simulink model "ModelVls"  (R2022b)
settings: Solver=FixedStepDiscrete  StartTime=0.0  StopTime=1  RelTol=1e-3  EnableMultiTasking=on
InitFcn:
  | % Initialize model
  | run([ModelRootName() 'Init.m']);
  | 
  | % load library data
  | GainLibrary_data;
StartFcn:
  | % make sure all the simulated RTC requests are found
  | %RTC_SIM_OBJ.ValidateREQs();
model workspace (MAT data in the model file):
  PreampVolumeTable_Idx : Simulink.Signal (value not decoded)
  Range : Simulink.Signal (value not decoded)
  Table_Idx : Simulink.Signal (value not decoded)
undefined symbols (not defined in the file): Config, Ifir, IFIR, MedusaConfig, MuteRamper, MuteRamperBtc, numAudioIn, preAmp, Row, sys_defs, VLSConfig
libraries: FeaturePath x22, TuneVar x17, RTC x9, MedusaDelays x9, dspindex x5, TOP x5, SampleRateConverter x4, EdgePorts x2, PooliirLib x2, MedusaCaeEnable x2, FIREven x2, VLSGains x2
(part 3 of 4)

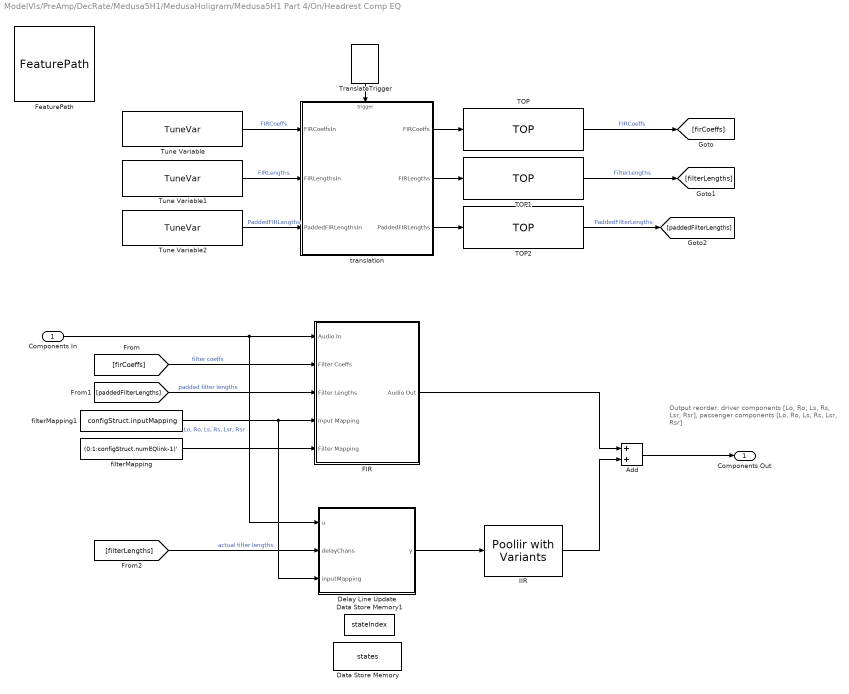
== system ModelVls/PreAmp/DecRate/Medusa5H1/MedusaHoligram/Medusa5H1 Part 4/On/Headrest Comp EQ ==
  note: Output reorder:
      | driver components [Lo, Ro, Ls, Rs, Lsr, Rsr],
      | passenger components [Lo, Ro, Ls, Rs, Lsr, Rsr]
  Components In : Inport
  Add : Sum  Priority=2
  Data Store Memory : DataStoreMemory  DataStoreName=states  ReadBeforeWriteMsg=warning  WriteAfterWriteMsg=warning  WriteAfterReadMsg=warning  InitialValue=zeros(fixedDelayLength, numInput)  ShowAdditionalParam=off  OutDataTypeStr=single
  Data Store Memory1 : DataStoreMemory  DataStoreName=stateIndex  ReadBeforeWriteMsg=warning  WriteAfterWriteMsg=warning  WriteAfterReadMsg=warning  ShowAdditionalParam=off  OutDataTypeStr=int32
  Delay Line Update : MATLAB Function  TreatAsAtomicUnit=on
  FIR : Subsystem  AncestorBlock=FIRGeneric/Generic FIR  mask(FIR Generic){variantSelect=Hexagon, stateBufferSize=configStruct.totalBufferSize, numOut=configStruct.numEQlink, frameSize=0, numIn=0}
      mask prompts: variantSelect "Implementation:"; stateBufferSize "State buffer size:"; numOut "Number of outputs:"; frameSize "Frame size:"; numIn "Number of inputs:"
      mask help:
      | Generic FIR is a configurable multi-channel FIR filter that supports one or more channels.  Different filter coefficients and number of coefficients can be used for each channel filter.  There can be fewer inputs than outputs, with some inputs routed to more than one output filter.   Identical filter configurations can also be used for multiple output filters.  The Generic FIR model supports three different implementations, selectable from the model mask:
      |
      | (i)  Core: FIR filters executing on core with target specific CRL support
      | (ii) Accel: FIR filters executing on IIR hardware accelerator, offloading MIPS usage from core
      | (iii) Hexagon: FIR filters executing on Hexagon DSP
      | (iv) Generic: FIR filters executing on core without CRL support
      |
      | NOTE: The Generic FIR codeWorkMemory buffer should always be mapped to L1 memory or core MIPS usage will increase.
      |
      | For more information, please see 'Help'.
      mask init:
      | % Create alias for code work memory buffer for each instance of model
      | FirGenericMask(gcbh, variantSelect);
      | 
      | % There are three implementation types:
      | % Type    Value  Description
      | % CORE    1      Optimized assembly running on core
      | % ACCEL   2      Computing offloaded to accelerator peripheral
      | % HEXAGON 3      Optimized C/assembly code running on Hexagon DSP
      | % GENERIC 4      Generic implementation for other targets without CRL
      | 
      | if variantSelect == 1
      |     % 6 variable size arrays (for input, coeffs, states, 
      |     % stateSharingEnabled, taps array per output channel,
      |     % and mapped audio input offsets) 
      |     % + 10 struct members
      |     codeWorkMemorySize = numOut * 6 + 10;  % words
      |     
      | elseif variantSelect == 2
      |     % Accelerator CRL code work memory size is equal to:
      |     %             sizeof(accelWorkMemory_t) + variableDataSize;
      |     % with variable data size dependent on number inputs, number outputs
      |     % and frame size.  NOTE: this must be updated to match the CRL code
      |     % if any changes are made to the accelWorkMemory_t structure.
      |     codeWorkMemorySize = 156 + (24 + numIn*48 + numOut*40);  % bytes
      |     codeWorkMemorySize = codeWorkMemorySize / 4;  % words (single)
      | 
      | elseif variantSelect == 3    
      |     codeWorkMemorySize = 156 + (24 + numIn*8 + numOut*(80 + 4*frameSize));  % bytes
      |     codeWorkMemorySize = codeWorkMemorySize / 4;  % words (single)
      |     
      | else
      |     % This is not used if there is no CRL
      |     codeWorkMemorySize = 1;
      | end
      settings: LibrarySourceBlock=FIRGeneric/Generic FIR
      mask Help:
      | Generic multi-channel FIR block supports multiple inputs, outputs and coefficient sets. Some inputs may drive multiple outputs, and this input sharing is specified by an input mapping per output. Some filters may be shared among multiple outputs, and this filter sharing is specified by a filter mapping per output. Input sharing assumes all filters sharing the same input have the same length to support state buffer sharing.
      | 
      | <b>Input signals: </b>
      | u: input channels [frame size x number of inputs]
      | coeffs: coefficient sets [total sum of filter lengths x 1]
      | filterLengths: array of filter lengths [number of filters x 1]
      | inputMapping: zero-based input mapping for each output [number of outputs x 1]
      | filterMapping:  zero-based filter mapping for each output [number of outputs x 1]
      | 
      | <b>Output signals: </b>
      | y: output channels [frame size x number of outputs]
      | 
      | <b>Mask parameters: </b>
      | Implementation: Core/Accel /Generic
      | State buffer size: total size of state buffer [total state buffer size x 1]
      | Number of outputs
      | Frame size
      | Number of inputs
      mask TypeOptions variantSelect: Core | Accel | Hexagon | Generic
      mask Callback variantSelect:
      | % Get the mask parameter value
      | maskStr = get_param(gcb,'variantSelect');
      | 
      | % Check the value of 'variantSelect'
      | if (~strcmp(maskStr,"Accel"))
      |     % Turn the visibility of 'frameSize' and 'numChannels' OFF
      |     set_param(gcb,'MaskVisibilities',{'on';'on';'on';'off';'off'});
      | else
      |     % "Accel": Set the visibility of all parameters to ON
      |     set_param(gcb,'MaskVisibilities',{'on';'on';'on';'on';'on'});
      | end
  FeaturePath : FeaturePath/FeaturePath  FeatureName=HeadrestCompEQ  IsGroup=off  GroupNumber=-1  IsModule=off  TriggerInit=[175 204 290 311]
      settings: SourceProductName=Bose Talaria
  IIR : PooliirAccel/Pooliir with Variants  variantSelect=Hexagon  maxNumStages=IIR.maxNumStages  numStages=IIR.numStages  sosCoefficients=IIR.coeffs  frameSize=0  numChannels=0  FeatureName=IIR
  TOP : TOP/TOP  TriggerInit=[815 320 985 380]  TopName=FIRCoeffs  DataType=single  BankNumber=1  PreOverlay=false  PostOverlay=false  Role=Automatic
      settings: SourceProductName=Bose Talaria
  TOP1 : TOP/TOP  TriggerInit=[815 390 985 450]  TopName=FilterLengths  DataType=uint32  BankNumber=0  PreOverlay=false  PostOverlay=false  Role=Automatic
      settings: SourceProductName=Bose Talaria
  TOP2 : TOP/TOP  TriggerInit=[815 460 985 520]  TopName=PaddedFilterLengths  DataType=uint32  BankNumber=0  PreOverlay=false  PostOverlay=false  Role=Automatic
      settings: SourceProductName=Bose Talaria
  TranslateTrigger : TuneVar/TranslateTrigger  TriggerInit=[656 230 694 285]
      settings: SourceProductName=Bose Talaria
  Tune Variable : TuneVar/TuneVar  TuneName=FIRCoeffs  SpecifyMaxSize=off  VariableDim=1 (Row)  MaxSize=[firLength*numEQlink 1]  TunabilityNumber=1  MinValue=[]  MaxValue=[]  TriggerInit=[330 325 500 375]  MaskValue=firCoeffsDefault
      settings: SourceProductName=Bose Talaria
  Tune Variable1 : TuneVar/TuneVar  TuneName=FIRLengths  SpecifyMaxSize=off  VariableDim=1 (Row)  MaxSize=[1 1]  TunabilityNumber=1  MinValue=[]  MaxValue=[]  TriggerInit=[330 395 500 445]  MaskValue=firLength*ones(numEQlink,1)
      settings: SourceProductName=Bose Talaria
  Tune Variable2 : TuneVar/TuneVar  TuneName=PaddedFIRLengths  SpecifyMaxSize=off  VariableDim=1 (Row)  MaxSize=[1 1]  TunabilityNumber=1  MinValue=[]  MaxValue=[]  TriggerInit=[330 465 500 515]  MaskValue=firLength*ones(numEQlink,1)
      settings: SourceProductName=Bose Talaria
  filterMapping : Constant  Value=(0:1:configStruct.numEQlink-1)'  VectorParams1D=off  OutDataTypeStr=uint32
  filterMapping1 : Constant  Value=configStruct.inputMapping  VectorParams1D=off  OutDataTypeStr=uint32
  translation : MATLAB Function  TreatAsAtomicUnit=on
  Components Out : Outport  VectorParamsAs1DForOutWhenUnconnected=off
  wires:
  Add/1 -> Components Out/1
  [firCoeffs] -> FIR/2(Filter Coeffs)  "filter coeffs"
  FIR/1(Audio Out) -> Add/1
  translation/2(FIRLengths) -> TOP1/1
  IIR/1 -> Add/2
  Tune Variable1/1 -> translation/2(FIRLengthsIn)  "FIRLengths"
  TOP/1 -> [firCoeffs]  "FIRCoeffs"
  filterMapping/1 -> FIR/5(Filter Mapping)
  translation/1(FIRCoeffs) -> TOP/1
  Delay Line Update/1(y) -> IIR/1
  TranslateTrigger/1 -> translation/Trigger
  Tune Variable/1 -> translation/1(FIRCoeffsIn)  "FIRCoeffs"
  filterMapping1/1 -> FIR/4(Input Mapping), Delay Line Update/3(inputMapping)
  [paddedFilterLengths] -> FIR/3(Filter Lengths)  "padded filter lengths"
  TOP1/1 -> [filterLengths]  "FilterLengths"
  Components In/1 -> FIR/1(Audio In), Delay Line Update/1(u)  "Lo, Ro, Ls, Rs, Lsr, Rsr"
  Tune Variable2/1 -> translation/3(PaddedFIRLengthsIn)  "PaddedFIRLengths"
  TOP2/1 -> [paddedFilterLengths]  "PaddedFilterLengths"
  translation/3(PaddedFIRLengths) -> TOP2/1
  [filterLengths] -> Delay Line Update/2(delayChans)  "actual filter lengths"

== system ModelVls/PreAmp/DecRate/Medusa5H1/PreAmpPart2/MuteRamperDR/InnerLink/Ramping_Subsystem ==
  audioIn : Inport
  Cg : Inport  Port=2
  Tg : Inport  Port=3
  RampCoeffs : Inport  Port=4
  SnapThresh : Inport  Port=5
  RampingGain : Subsystem
  Variable Selector : dspindex/Variable Selector  NumInputs=1  rowsOrCols=Rows  IdxMode=Fixed  Elements=Config.SamplesPerFrame  ZerOneIdxMode=One-based  errmode=Clip Index  FillMode=on  FillValues=0
  applyGain : Subsystem
  Out : Outport  VectorParamsAs1DForOutWhenUnconnected=off
  current_gain : Outport  Port=2  VectorParamsAs1DForOutWhenUnconnected=off
  wires:
  RampCoeffs/1 -> RampingGain/3(RampCoeffs)
  Tg/1 -> RampingGain/2(TargetGain)
  SnapThresh/1 -> RampingGain/4(SnapThresh)
  Cg/1 -> RampingGain/1(CurrentGain)
  Variable Selector/1 -> current_gain/1
  applyGain/1(Out1) -> Out/1
  audioIn/1 -> applyGain/2(In2)
  RampingGain/1(current_gain_out) -> Variable Selector/1, applyGain/1(In1)

== system ModelVls/PreAmp/DecRate/Medusa5H1/PreAmpPart2/MuteRamperFR/InnerLink/Ramping_Subsystem ==
  audioIn : Inport
  Cg : Inport  Port=2
  Tg : Inport  Port=3
  RampCoeffs : Inport  Port=4
  SnapThresh : Inport  Port=5
  RampingGain : Subsystem
  Variable Selector : dspindex/Variable Selector  NumInputs=1  rowsOrCols=Rows  IdxMode=Fixed  Elements=Config.SamplesPerFrame  ZerOneIdxMode=One-based  errmode=Clip Index  FillMode=on  FillValues=0
  applyGain : Subsystem
  Out : Outport  VectorParamsAs1DForOutWhenUnconnected=off
  current_gain : Outport  Port=2  VectorParamsAs1DForOutWhenUnconnected=off
  wires:
  RampCoeffs/1 -> RampingGain/3(RampCoeffs)
  Tg/1 -> RampingGain/2(TargetGain)
  SnapThresh/1 -> RampingGain/4(SnapThresh)
  Cg/1 -> RampingGain/1(CurrentGain)
  Variable Selector/1 -> current_gain/1
  applyGain/1(Out1) -> Out/1
  audioIn/1 -> applyGain/2(In2)
  RampingGain/1(current_gain_out) -> Variable Selector/1, applyGain/1(In1)

== system ModelVls/PreAmp/DecRate/Medusa5H1/MedusaHoligram/Medusa5H1 Part 3/On/SLC/Merge NTF_done ==
  NTF_done_DR : Inport
  NTF_done_FR : Inport  Port=2
  NTF_done_DR_VLS : Inport  Port=3
  NTF_done_FR_VLS : Inport  Port=4
  Trigger : TriggerPort  TriggerType=function-call  VariantControl=Variant  PortDimensions=1
  AND : Logic  Inputs=4  IconShape=distinctive  AllPortsSameDT=off  OutDataTypeStr=boolean
  NTF_done : Outport  VectorParamsAs1DForOutWhenUnconnected=off
  wires:
  NTF_done_FR_VLS/1 -> AND/4
  NTF_done_DR_VLS/1 -> AND/3
  NTF_done_DR/1 -> AND/1
  NTF_done_FR/1 -> AND/2
  AND/1 -> NTF_done/1

== system ModelVls/PreAmp/DecRate/Medusa5H1/MedusaHoligram/Medusa5H1 Part 4/On/Headrest Comp EQ/FIR ==
  Audio In : Inport
  Filter Coeffs : Inport  Port=2
  Filter Lengths : Inport  Port=3
  Input Mapping : Inport  Port=4
  Filter Mapping : Inport  Port=5
  FIR generic init : MATLAB Function  TreatAsAtomicUnit=on  RTWFcnName=foo
  FeaturePath : FeaturePath/FeaturePath  FeatureName=FIR  IsGroup=off  GroupNumber=-1  IsModule=off  TriggerInit=[105 -141 220 -34]
      settings: SourceProductName=Bose Talaria
  ITC : Subsystem  mask(Bose Initialization Trigger Control){}
      mask help: This block emits a function trigger for logic intended to execute at subsystem initialization time. Make sure not to reference any "live" signals
      mask init:
      | CodeID = InitTriggerControlMask.DoInit(gcbh);
      | ok = true;
      mask Display:
      | % retrieve icon definition
      | [path,w,h] = InitTriggerControlMask.Icon();
      | 
      | % retrieve the block's pixel size
      | pos = get(gcbh,'position');
      | bw = pos(3) - pos(1);
      | bh = pos(4) - pos(2);
      | 
      | % draw  icon to the center left
      | xAdj = bw/2 - w/2;
      | yAdj = bh/2 - h/2 + 4;
      | for i=1:length(path)
      |     patch(path(i).x+xAdj, path(i).y+yAdj, path(i).rgb);
      | end
      | 
      | text(bw*0.5, bh*0.2, 'ITC', 'horizontalAlignment', 'center');
      | 
      | % show X on error
      | if (exist('ok','var') && ok)
      | 	patch(0,0,[1 1 1]);
      | 	patch(bw,bh,[1 1 1]);
      | else
      | 	tx=bw*0.03;
      | 	ty=bh*0.03;
      | 	patch([0 tx bw bw-tx], [ty 0 bh-ty bh], [1 0 0]);
      | 	patch([0 bw-tx bw tx], [bh-ty 0 ty bh], [1 0 0]);
      | end
  MATLAB Function : MATLAB Function  TreatAsAtomicUnit=on
  codeWorkMemory : DataStoreMemory  DataStoreName=codeWorkMemory  WriteAfterWriteMsg=warning  InitialValue=zeros(1,codeWorkMemorySize)  ShowAdditionalParam=off  OutDataTypeStr=uint32
  stateBuffer : DataStoreMemory  DataStoreName=states  ReadBeforeWriteMsg=warning  WriteAfterWriteMsg=warning  WriteAfterReadMsg=warning  InitialValue=zeros(stateBufferSize,1)  ShowAdditionalParam=off  OutDataTypeStr=single
  Audio Out : Outport  VectorParamsAs1DForOutWhenUnconnected=off
  wires:
  Audio In/1 -> MATLAB Function/1(u), FIR generic init/1(u)
  ITC/1(Out1) -> FIR generic init/Trigger
  MATLAB Function/1(y) -> Audio Out/1
  Filter Mapping/1 -> MATLAB Function/5(filterMapping), FIR generic init/5(filterMapping)
  Filter Coeffs/1 -> MATLAB Function/2(coeffs), FIR generic init/2(coeffs)
  Input Mapping/1 -> MATLAB Function/4(inputMapping), FIR generic init/4(inputMapping)
  Filter Lengths/1 -> MATLAB Function/3(filterLengths), FIR generic init/3(filterLengths)

== system ModelVls/PreAmp/DecRate/Medusa5H1/PreAmpPart2/MuteRamperDR/InnerLink/Ramping_Subsystem/RampingGain ==
  CurrentGain : Inport
  TargetGain : Inport  Port=2
  RampCoeffs : Inport  Port=3
  SnapThresh : Inport  Port=4
  Abs3 : Abs  SaturateOnIntegerOverflow=off
  Add : Sum  Inputs=+-
  If : If  NumInputs=3  IfExpression=(u1>u2) & (u3>0)
  Max : MinMax  Function=max  Inputs=2
  Merge : Merge
  elseActionSubsystem : Subsystem
  frames : DataStoreRead  DataStoreName=nFrames  IndexOptions=Index vector (dialog)  Indices=1  OutputSizes=1
  ifActionSubsystem : Subsystem
  minGain : Constant  Value=Config.SilentGainLinear  OutDataTypeStr=single
  current_gain_out : Outport  VectorParamsAs1DForOutWhenUnconnected=off
  wires:
  frames/1 -> If/3, ifActionSubsystem/4(nFrames)
  elseActionSubsystem/1(Out1) -> Merge/2
  ifActionSubsystem/1(Out1) -> Merge/1
  RampCoeffs/1 -> ifActionSubsystem/1(rampCoeff)
  If/2 -> elseActionSubsystem/Action
  If/1 -> ifActionSubsystem/Action
  CurrentGain/1 -> Max/1
  minGain/1 -> Max/2
  Abs3/1 -> If/1
  SnapThresh/1 -> If/2
  TargetGain/1 -> elseActionSubsystem/1(In1), Add/1, ifActionSubsystem/2(TargetGain)
  Add/1 -> Abs3/1
  Merge/1 -> current_gain_out/1
  Max/1 -> Add/2, ifActionSubsystem/3(CurrentGain)

== system ModelVls/PreAmp/DecRate/Medusa5H1/PreAmpPart2/MuteRamperDR/InnerLink/Ramping_Subsystem/applyGain ==
  In1 : Inport
  In2 : Inport  Port=2
  For Each Subsystem : Subsystem  TreatAsAtomicUnit=on
  Out1 : Outport  VectorParamsAs1DForOutWhenUnconnected=off
  wires:
  In1/1 -> For Each Subsystem/1(In1)
  For Each Subsystem/1(Out1) -> Out1/1
  In2/1 -> For Each Subsystem/2(In2)

== system ModelVls/PreAmp/DecRate/Medusa5H1/PreAmpPart2/MuteRamperFR/InnerLink/Ramping_Subsystem/RampingGain ==
  CurrentGain : Inport
  TargetGain : Inport  Port=2
  RampCoeffs : Inport  Port=3
  SnapThresh : Inport  Port=4
  Abs3 : Abs  SaturateOnIntegerOverflow=off
  Add : Sum  Inputs=+-
  If : If  NumInputs=3  IfExpression=(u1>u2) & (u3>0)
  Max : MinMax  Function=max  Inputs=2
  Merge : Merge
  elseActionSubsystem : Subsystem
  frames : DataStoreRead  DataStoreName=nFrames  IndexOptions=Index vector (dialog)  Indices=1  OutputSizes=1
  ifActionSubsystem : Subsystem
  minGain : Constant  Value=Config.SilentGainLinear  OutDataTypeStr=single
  current_gain_out : Outport  VectorParamsAs1DForOutWhenUnconnected=off
  wires:
  frames/1 -> If/3, ifActionSubsystem/4(nFrames)
  elseActionSubsystem/1(Out1) -> Merge/2
  ifActionSubsystem/1(Out1) -> Merge/1
  RampCoeffs/1 -> ifActionSubsystem/1(rampCoeff)
  If/2 -> elseActionSubsystem/Action
  If/1 -> ifActionSubsystem/Action
  CurrentGain/1 -> Max/1
  minGain/1 -> Max/2
  Abs3/1 -> If/1
  SnapThresh/1 -> If/2
  TargetGain/1 -> elseActionSubsystem/1(In1), Add/1, ifActionSubsystem/2(TargetGain)
  Add/1 -> Abs3/1
  Merge/1 -> current_gain_out/1
  Max/1 -> Add/2, ifActionSubsystem/3(CurrentGain)

== system ModelVls/PreAmp/DecRate/Medusa5H1/PreAmpPart2/MuteRamperFR/InnerLink/Ramping_Subsystem/applyGain ==
  In1 : Inport
  In2 : Inport  Port=2
  For Each Subsystem : Subsystem  TreatAsAtomicUnit=on
  Out1 : Outport  VectorParamsAs1DForOutWhenUnconnected=off
  wires:
  In1/1 -> For Each Subsystem/1(In1)
  For Each Subsystem/1(Out1) -> Out1/1
  In2/1 -> For Each Subsystem/2(In2)

== system ModelVls/PreAmp/DecRate/Medusa5H1/MedusaHoligram/Medusa5H1 Part 4/On/Headrest Comp EQ/FIR/ITC ==
  ITC1 : S-Function  FunctionName=InitTriggerControl  Parameters=CodeID, 0  SFunctionDeploymentMode=off  EnableBusSupport=off
  init : MATLAB Function  TreatAsAtomicUnit=on  RTWFcnName=InitTrigger_Model_4079_595_209_62
      settings: RTWSystemCode=Nonreusable function
  Out1 : Outport  VectorParamsAs1DForOutWhenUnconnected=off
  wires:
  init/1(init()) -> Out1/1
  ITC1/1 -> init/Trigger

== system ModelVls/PreAmp/DecRate/Medusa5H1/PreAmpPart2/MuteRamperDR/InnerLink/Ramping_Subsystem/RampingGain/elseActionSubsystem ==
  In1 : Inport
  Action Port : ActionPort  ActionPortLabel=else
  Constant : Constant  Value=ones(Config.SamplesPerFrame,1)  VectorParams1D=off  OutDataTypeStr=single
  Multiply : Product
  Out1 : Outport  VectorParamsAs1DForOutWhenUnconnected=off
  wires:
  Constant/1 -> Multiply/1
  In1/1 -> Multiply/2
  Multiply/1 -> Out1/1

== system ModelVls/PreAmp/DecRate/Medusa5H1/PreAmpPart2/MuteRamperDR/InnerLink/Ramping_Subsystem/RampingGain/ifActionSubsystem ==
  note: IIR filter is used to get ramping up/down gain values. Filter transfer function
      |  is calculated for equation:
      | 	gain(n) = gain(n-1)*ramp_coeff
      |
      | Denominator coeff  = [1, -rampcoeff]  and Numerator coeff = 0
      | x0 : Initial state of the filter which is (currentGain * rampCoeff)
      | III : When target gain is updated through RTC, this signal will reset filter to
      | 	initial state to serve new RTC request
  rampCoeff : Inport
  TargetGain : Inport  Port=2
  CurrentGain : Inport  Port=3
  nFrames : Inport  Port=4
  Action Port : ActionPort  ActionPortLabel=if((u1>u2) & (u3>0))
  Add : Sum  Inputs=+-
  Constant : Constant  Value=ones(Config.SamplesPerFrame,1)  VectorParams1D=off  OutDataTypeStr=single
  Constant1 : Constant  OutDataTypeStr=single
  Data Store Write : DataStoreWrite  DataStoreName=nFrames  IndexOptions=Index vector (dialog)  Indices=1  OutputSizes=1
  Matrix Multiply : Product
  denCoefficient : Subsystem
  ramping_filter : DiscreteFilter  Numerator=0  DenominatorSource=Input port  Denominator=[1 -1.0003]  InitialStatesSource=Input port  InitialStates=1.0003  InputProcessing=Columns as channels (frame based)  ExternalReset=Level hold  FilterStructure=Direct form II transposed  a0EqualsOne=on
      settings: InputPortMap=u0,p3,r7,p5
  resetFilter : Subsystem
  Out1 : Outport
  wires:
  nFrames/1 -> Add/1
  Constant1/1 -> Add/2
  Add/1 -> Data Store Write/1
  Matrix Multiply/1 -> ramping_filter/4
  CurrentGain/1 -> Matrix Multiply/2
  ramping_filter/1 -> Out1/1
  Constant/1 -> ramping_filter/1
  rampCoeff/1 -> Matrix Multiply/1, denCoefficient/1(In1)
  resetFilter/1(Out1) -> ramping_filter/3
  denCoefficient/1(Out1) -> ramping_filter/2
  TargetGain/1 -> resetFilter/1(In1)

== system ModelVls/PreAmp/DecRate/Medusa5H1/PreAmpPart2/MuteRamperDR/InnerLink/Ramping_Subsystem/applyGain/For Each Subsystem ==
  In1 : Inport  Partition=on  PartitionDimension=1  PartitionWidth=1  PartitionOffset=0
  In2 : Inport  Port=2  Partition=on  PartitionDimension=1  PartitionWidth=1  PartitionOffset=0
  For Each : ForEach  DisableCoverage=on
  Multiply : Product  Multiplication=Matrix(*)
  Out1 : Outport  ConcatenationDimension=1
  wires:
  Multiply/1 -> Out1/1
  In2/1 -> Multiply/2
  In1/1 -> Multiply/1

== system ModelVls/PreAmp/DecRate/Medusa5H1/PreAmpPart2/MuteRamperFR/InnerLink/Ramping_Subsystem/RampingGain/elseActionSubsystem ==
  In1 : Inport
  Action Port : ActionPort  ActionPortLabel=else
  Constant : Constant  Value=ones(Config.SamplesPerFrame,1)  VectorParams1D=off  OutDataTypeStr=single
  Multiply : Product
  Out1 : Outport  VectorParamsAs1DForOutWhenUnconnected=off
  wires:
  Constant/1 -> Multiply/1
  In1/1 -> Multiply/2
  Multiply/1 -> Out1/1

== system ModelVls/PreAmp/DecRate/Medusa5H1/PreAmpPart2/MuteRamperFR/InnerLink/Ramping_Subsystem/RampingGain/ifActionSubsystem ==
  note: IIR filter is used to get ramping up/down gain values. Filter transfer function
      |  is calculated for equation:
      | 	gain(n) = gain(n-1)*ramp_coeff
      |
      | Denominator coeff  = [1, -rampcoeff]  and Numerator coeff = 0
      | x0 : Initial state of the filter which is (currentGain * rampCoeff)
      | III : When target gain is updated through RTC, this signal will reset filter to
      | 	initial state to serve new RTC request
  rampCoeff : Inport
  TargetGain : Inport  Port=2
  CurrentGain : Inport  Port=3
  nFrames : Inport  Port=4
  Action Port : ActionPort  ActionPortLabel=if((u1>u2) & (u3>0))
  Add : Sum  Inputs=+-
  Constant : Constant  Value=ones(Config.SamplesPerFrame,1)  VectorParams1D=off  OutDataTypeStr=single
  Constant1 : Constant  OutDataTypeStr=single
  Data Store Write : DataStoreWrite  DataStoreName=nFrames  IndexOptions=Index vector (dialog)  Indices=1  OutputSizes=1
  Matrix Multiply : Product
  denCoefficient : Subsystem
  ramping_filter : DiscreteFilter  Numerator=0  DenominatorSource=Input port  Denominator=[1 -1.0003]  InitialStatesSource=Input port  InitialStates=1.0003  InputProcessing=Columns as channels (frame based)  ExternalReset=Level hold  FilterStructure=Direct form II transposed  a0EqualsOne=on
      settings: InputPortMap=u0,p3,r7,p5
  resetFilter : Subsystem
  Out1 : Outport
  wires:
  nFrames/1 -> Add/1
  Constant1/1 -> Add/2
  Add/1 -> Data Store Write/1
  Matrix Multiply/1 -> ramping_filter/4
  CurrentGain/1 -> Matrix Multiply/2
  ramping_filter/1 -> Out1/1
  Constant/1 -> ramping_filter/1
  rampCoeff/1 -> Matrix Multiply/1, denCoefficient/1(In1)
  resetFilter/1(Out1) -> ramping_filter/3
  denCoefficient/1(Out1) -> ramping_filter/2
  TargetGain/1 -> resetFilter/1(In1)

== system ModelVls/PreAmp/DecRate/Medusa5H1/PreAmpPart2/MuteRamperFR/InnerLink/Ramping_Subsystem/applyGain/For Each Subsystem ==
  In1 : Inport  Partition=on  PartitionDimension=1  PartitionWidth=1  PartitionOffset=0
  In2 : Inport  Port=2  Partition=on  PartitionDimension=1  PartitionWidth=1  PartitionOffset=0
  For Each : ForEach  DisableCoverage=on
  Multiply : Product  Multiplication=Matrix(*)
  Out1 : Outport  ConcatenationDimension=1
  wires:
  Multiply/1 -> Out1/1
  In2/1 -> Multiply/2
  In1/1 -> Multiply/1

== system ModelVls/PreAmp/DecRate/Medusa5H1/PreAmpPart2/MuteRamperDR/InnerLink/Ramping_Subsystem/RampingGain/ifActionSubsystem/denCoefficient ==
  In1 : Inport
  Constant : Constant  Value=-1  OutDataTypeStr=single
  Constant3 : Constant  OutDataTypeStr=single
  Matrix Concatenate : Concatenate  Mode=Multidimensional array  ConcatenateDimension=2
  Multiply : Product
  Out1 : Outport  VectorParamsAs1DForOutWhenUnconnected=off
  wires:
  In1/1 -> Multiply/2
  Multiply/1 -> Matrix Concatenate/2
  Constant/1 -> Multiply/1
  Matrix Concatenate/1 -> Out1/1
  Constant3/1 -> Matrix Concatenate/1

== system ModelVls/PreAmp/DecRate/Medusa5H1/PreAmpPart2/MuteRamperDR/InnerLink/Ramping_Subsystem/RampingGain/ifActionSubsystem/resetFilter ==
  In1 : Inport
  Add2 : Sum  Inputs=+-
  Delay : Delay  DelayLength=1
  If : If  IfExpression=u1 == 0
  If Action Subsystem : Subsystem  TreatAsAtomicUnit=on
  If Action Subsystem1 : Subsystem  TreatAsAtomicUnit=on
  Merge : Merge
  Out1 : Outport  VectorParamsAs1DForOutWhenUnconnected=off
  wires:
  Merge/1 -> Out1/1
  If Action Subsystem1/1(Out1) -> Merge/2
  If Action Subsystem/1(Out1) -> Merge/1
  If/2 -> If Action Subsystem1/Action
  If/1 -> If Action Subsystem/Action
  In1/1 -> Delay/1, Add2/1
  Delay/1 -> Add2/2
  Add2/1 -> If/1

== system ModelVls/PreAmp/DecRate/Medusa5H1/PreAmpPart2/MuteRamperFR/InnerLink/Ramping_Subsystem/RampingGain/ifActionSubsystem/denCoefficient ==
  In1 : Inport
  Constant : Constant  Value=-1  OutDataTypeStr=single
  Constant3 : Constant  OutDataTypeStr=single
  Matrix Concatenate : Concatenate  Mode=Multidimensional array  ConcatenateDimension=2
  Multiply : Product
  Out1 : Outport  VectorParamsAs1DForOutWhenUnconnected=off
  wires:
  In1/1 -> Multiply/2
  Multiply/1 -> Matrix Concatenate/2
  Constant/1 -> Multiply/1
  Matrix Concatenate/1 -> Out1/1
  Constant3/1 -> Matrix Concatenate/1

== system ModelVls/PreAmp/DecRate/Medusa5H1/PreAmpPart2/MuteRamperFR/InnerLink/Ramping_Subsystem/RampingGain/ifActionSubsystem/resetFilter ==
  In1 : Inport
  Add2 : Sum  Inputs=+-
  Delay : Delay  DelayLength=1
  If : If  IfExpression=u1 == 0
  If Action Subsystem : Subsystem  TreatAsAtomicUnit=on
  If Action Subsystem1 : Subsystem  TreatAsAtomicUnit=on
  Merge : Merge
  Out1 : Outport  VectorParamsAs1DForOutWhenUnconnected=off
  wires:
  Merge/1 -> Out1/1
  If Action Subsystem1/1(Out1) -> Merge/2
  If Action Subsystem/1(Out1) -> Merge/1
  If/2 -> If Action Subsystem1/Action
  If/1 -> If Action Subsystem/Action
  In1/1 -> Delay/1, Add2/1
  Delay/1 -> Add2/2
  Add2/1 -> If/1

== system ModelVls/PreAmp/DecRate/Medusa5H1/PreAmpPart2/MuteRamperDR/InnerLink/Ramping_Subsystem/RampingGain/ifActionSubsystem/resetFilter/If Action Subsystem ==
  Action Port : ActionPort  ActionPortLabel=if(u1 == 0)
  Constant : Constant  Value=0  OutDataTypeStr=boolean
  Out1 : Outport  VectorParamsAs1DForOutWhenUnconnected=off
  wires:
  Constant/1 -> Out1/1

== system ModelVls/PreAmp/DecRate/Medusa5H1/PreAmpPart2/MuteRamperDR/InnerLink/Ramping_Subsystem/RampingGain/ifActionSubsystem/resetFilter/If Action Subsystem1 ==
  Action Port : ActionPort  ActionPortLabel=else
  Constant : Constant  OutDataTypeStr=boolean
  Out1 : Outport  VectorParamsAs1DForOutWhenUnconnected=off
  wires:
  Constant/1 -> Out1/1

== system ModelVls/PreAmp/DecRate/Medusa5H1/PreAmpPart2/MuteRamperFR/InnerLink/Ramping_Subsystem/RampingGain/ifActionSubsystem/resetFilter/If Action Subsystem ==
  Action Port : ActionPort  ActionPortLabel=if(u1 == 0)
  Constant : Constant  Value=0  OutDataTypeStr=boolean
  Out1 : Outport  VectorParamsAs1DForOutWhenUnconnected=off
  wires:
  Constant/1 -> Out1/1

== system ModelVls/PreAmp/DecRate/Medusa5H1/PreAmpPart2/MuteRamperFR/InnerLink/Ramping_Subsystem/RampingGain/ifActionSubsystem/resetFilter/If Action Subsystem1 ==
  Action Port : ActionPort  ActionPortLabel=else
  Constant : Constant  OutDataTypeStr=boolean
  Out1 : Outport  VectorParamsAs1DForOutWhenUnconnected=off
  wires:
  Constant/1 -> Out1/1

== matlab function ModelVls/PreAmp/DecRate/Medusa5H1/MedusaHoligram/Medusa5H1 Part 4/On/Headrest Comp EQ/translation ==
  data: FIRCoeffs output; FIRCoeffsIn input; FIRLengths output; FIRLengthsIn input; PaddedFIRLengthsIn input; PaddedFIRLengths output
  events: trigger input FUNCTION_CALL_EVENT
function [FIRCoeffs, FIRLengths, PaddedFIRLengths] = fcn(FIRCoeffsIn, FIRLengthsIn, PaddedFIRLengthsIn)

FIRCoeffs = FIRCoeffsIn.Value;
FIRLengths = FIRLengthsIn.Value;
PaddedFIRLengths = PaddedFIRLengthsIn.Value;

== matlab function ModelVls/PreAmp/DecRate/Medusa5H1/PreAmpPart2/MuteRamperDR/InnerLink/TriggeredFunction ==
  data: done output; targetLinearGain data_store_memory; currentGain data_store_memory
  events: trigger input FUNCTION_CALL_EVENT
function done = NotificationCheck()
% Function to check whether the ramp has completed. 
% If so, send out TRUE

global targetLinearGain;
global currentGain;

% Assume the work is complete until proven otherwise
done = true;
if (targetLinearGain ~= currentGain)
   done = false; % just proved otherwise
end

== matlab function ModelVls/PreAmp/DecRate/Medusa5H1/PreAmpPart2/MuteRamperDR/InnerLink/get_ramp_coeffs ==
  data: currentGainValue input; muteSwitch input; ramping_coeff output; rampingRate_dBPerSec input; rampingTime_ms input; Fs_Hz input; silentGainLinear parameter; targetLinearGain data_store_memory; nFrames data_store_memory; frameSize parameter
  events: trigger input FUNCTION_CALL_EVENT
function ramping_coeff = fcn(currentGainValue, muteSwitch, rampingRate_dBPerSec,rampingTime_ms, Fs_Hz, silentGainLinear, frameSize)

global targetLinearGain
global nFrames
targetLinearGain = single(1.0);

if muteSwitch
    targetLinearGain = single(max(0, silentGainLinear));
end

% % Nudge the gain values a bit if they are sitting at zero.
% % If current gain is zero, replace with a value very close to zero. What we
% % really want is a value which is on the edge of perception - not too small
% % or large. If the value is too small, we'll waste some of our ramp time
% % in perceived silence. If the value is too large, the audio will lurch
% % into perceptability at the start of the ramp.
% % So, 'max(currentGainValue, silentGainLinear)' & 'max(TargetGain, silentGainLinear)' are
% % used in equations

% In order to have the desired ramp time, the slope must vary dependent
% on the gain difference between target and current value.
% Equivalent ramp rate is therefore calculated as follows:

if (rampingRate_dBPerSec)
    currentGain_db = 20*log10(max(currentGainValue, silentGainLinear));
    targetGain_db = 20*log10( targetLinearGain);
    diff = abs(currentGain_db - targetGain_db);
    rampingTime_ms = diff / single(rampingRate_dBPerSec) * 1000;
end

quantum_ms = 1000 * frameSize / Fs_Hz;
numFrames = rampingTime_ms / quantum_ms;
% Do a ceil rather than a round to insure that we create enough
% frames. i.e. a fraction of a frame is promoted to an addition frame
nFrames = max (1, ceil(numFrames));
quantized_rampTime_ms = nFrames * quantum_ms;
   
% In order to have the desired ramp time, the slope must vary dependent
% on the gain differencebetween target and current value.
% Ramper's coefficient is therefore calculated as follows:
%
%   TargetGain = CurrentGain *( RampCoef ^ (Fs*RampTime_ms/1000) )
%
% therefore...
%
%                     log(TargetGain/CurrentGain)
%   log(RampCoef) = ------------------------------
%                        Fs*(RampTime_ms/1000)
%
ramping_coeff= exp(log( targetLinearGain /max(currentGainValue, silentGainLinear) ) / (Fs_Hz * quantized_rampTime_ms / 1000));

== matlab function ModelVls/PreAmp/DecRate/Medusa5H1/PreAmpPart2/MuteRamperFR/InnerLink/TriggeredFunction ==
  data: done output; targetLinearGain data_store_memory; currentGain data_store_memory
  events: trigger input FUNCTION_CALL_EVENT
function done = NotificationCheck()
% Function to check whether the ramp has completed. 
% If so, send out TRUE

global targetLinearGain;
global currentGain;

% Assume the work is complete until proven otherwise
done = true;
if (targetLinearGain ~= currentGain)
   done = false; % just proved otherwise
end

== matlab function ModelVls/PreAmp/DecRate/Medusa5H1/PreAmpPart2/MuteRamperFR/InnerLink/get_ramp_coeffs ==
  data: currentGainValue input; muteSwitch input; ramping_coeff output; rampingRate_dBPerSec input; rampingTime_ms input; Fs_Hz input; silentGainLinear parameter; targetLinearGain data_store_memory; nFrames data_store_memory; frameSize parameter
  events: trigger input FUNCTION_CALL_EVENT
function ramping_coeff = fcn(currentGainValue, muteSwitch, rampingRate_dBPerSec,rampingTime_ms, Fs_Hz, silentGainLinear, frameSize)

global targetLinearGain
global nFrames
targetLinearGain = single(1.0);

if muteSwitch
    targetLinearGain = single(max(0, silentGainLinear));
end

% % Nudge the gain values a bit if they are sitting at zero.
% % If current gain is zero, replace with a value very close to zero. What we
% % really want is a value which is on the edge of perception - not too small
% % or large. If the value is too small, we'll waste some of our ramp time
% % in perceived silence. If the value is too large, the audio will lurch
% % into perceptability at the start of the ramp.
% % So, 'max(currentGainValue, silentGainLinear)' & 'max(TargetGain, silentGainLinear)' are
% % used in equations

% In order to have the desired ramp time, the slope must vary dependent
% on the gain difference between target and current value.
% Equivalent ramp rate is therefore calculated as follows:

if (rampingRate_dBPerSec)
    currentGain_db = 20*log10(max(currentGainValue, silentGainLinear));
    targetGain_db = 20*log10( targetLinearGain);
    diff = abs(currentGain_db - targetGain_db);
    rampingTime_ms = diff / single(rampingRate_dBPerSec) * 1000;
end

quantum_ms = 1000 * frameSize / Fs_Hz;
numFrames = rampingTime_ms / quantum_ms;
% Do a ceil rather than a round to insure that we create enough
% frames. i.e. a fraction of a frame is promoted to an addition frame
nFrames = max (1, ceil(numFrames));
quantized_rampTime_ms = nFrames * quantum_ms;
   
% In order to have the desired ramp time, the slope must vary dependent
% on the gain differencebetween target and current value.
% Ramper's coefficient is therefore calculated as follows:
%
%   TargetGain = CurrentGain *( RampCoef ^ (Fs*RampTime_ms/1000) )
%
% therefore...
%
%                     log(TargetGain/CurrentGain)
%   log(RampCoef) = ------------------------------
%                        Fs*(RampTime_ms/1000)
%
ramping_coeff= exp(log( targetLinearGain /max(currentGainValue, silentGainLinear) ) / (Fs_Hz * quantized_rampTime_ms / 1000));

== matlab function ModelVls/PreAmp/DecRate/Medusa5H1/MedusaHoligram/Medusa5H1 Part 1/Medusa Band Split Stereo/Interpolated Filter/ifir ==
  data: audioIn input; coeffsFlip parameter; audioOut output; I parameter; states data_store_memory
function audioOut = ifir(audioIn, coeffsFlip, I)

% An interpolated FIR filter is an FIR filter with a sparse set of
% coefficients.  That is, the coefficients contain I-1 zeros between
% each point, so the effective length of  filter is len(input_coeffs) * I  
% The function support multiple channels, with each
% channel sharing the same set of filter coefficients.
% 
% p : coefficient set (non-zero coefficients)
% I : interpolation factor, I-1 zeros are inserted between each coefficient
% 
% NOTES: 
% The legacy IFIR block supported coefficient sets.  Currently
% this only supports one coefficient set. 
% The coefficients are stored flipped in time. The unflipped coeffs are
% passed to block mask, and the flipping is done in mask initialization.

% Initialize variables
[frameSize, numChannels] = size(audioIn);
[filterLength, ~] = size(coeffsFlip);

frameSize   = uint32(frameSize);
numChannels = uint32(numChannels);
filterLength = int32(filterLength);
activeCoeffSet = coder.const(uint32(zeros(1,numChannels)));

% State is a circular buffer that holds previous stateLen samples, 
% where state_index points to the last/oldest sample in the buffer, which 
% during processing will be overwritten by the current input sample.
global states;

persistent state_index;
if isempty(state_index)
    state_index = int32(0);
end

audioOut = IFIR(audioIn, frameSize, numChannels, states, filterLength, ...
                    state_index, coeffsFlip, activeCoeffSet, I);
                
end

function y = IFIR(audioIn, frameSize, numChannels, states2, filterLength, ...
                    state_index2, coeffsFlip, activeCoeffSet, I)
% If code gen'ing, generate warning if this is not replaced with IFIR.asm
%coder.replace('-warnifnoreplacement');

% We have to use a different state buffer and state index than the one 
% passed in.  Matlab value objects are passed by value, not by reference, 
% so the saving of states here does not work.  The state buffer and index 
% are still necessary to pass allocate in the calling function and pass 
% here in order to trigger CRL. This double buffering is annoying, however 
% only happens during simulation, not code generation. (taken from pooliir)
global states;
persistent state_index;
if isempty(state_index)
    state_index = int32(0);
end

y = coder.nullcopy(audioIn);
stateLen = filterLength * I;

for channel = 1:numChannels
    state = states(:,channel);
    stateIndex = state_index;
    coeffs = coeffsFlip(:,activeCoeffSet(channel)+1);
    
    for sample = 1:frameSize
        % overwrite oldest sample with the current input sample
        state(stateIndex+1) = audioIn(sample, channel);
        % go to the oldest sample (previously the 2nd oldest)
        stateIndex = stateIndex + I; 
        if (stateIndex >= stateLen)
            stateIndex = stateIndex - stateLen;
        end

        accum = single(0);
        for i = 1:filterLength
            accum = accum + (state(stateIndex+1) * coeffs(i));
            stateIndex = stateIndex + I; % skip zero coefficients
            if (stateIndex >= stateLen)
                    stateIndex = stateIndex - stateLen;
            end
        end
        y(sample, channel) = accum;

        % update stateIndex for next sample
        % because we subtract here state_index type is int32 not uint32
        stateIndex = stateIndex - (I-1);
        if (stateIndex < 0)
            stateIndex = stateIndex + stateLen;
        end
    end
 
    states(:, channel) = state;
end

state_index = stateIndex;

end

== matlab function ModelVls/NEAR/MATLAB Function ==
  data: u input; y output
function y = fcn(u)

y = u;

== matlab function ModelVls/PreAmp/Reset/MATLAB Function ==
  events: trigger input FUNCTION_CALL_EVENT
function fcn()

if coder.target('Rtw')
    coder.ceval('Model_Target_DRFDP_initialize');
    coder.ceval('Model_Target_FRFDP_initialize');
    coder.ceval('Model_Target_ExpandTailComponents_initialize');
    coder.ceval('Model_Target_TrebleandSurroundDelays_initialize');
    coder.ceval('Model_Target_Medusa5H1Part3_initialize');
    coder.ceval('Model_Target_Subsystem_initialize');
    
    coder.ceval('Model_Target_PreAmpPart1_Start');
    coder.ceval('Model_Target_SRCIn_Start');
%     coder.ceval('Model_Target_AudioPilot35_Start');
    coder.ceval('Model_Target_Medusa5H1Part1_Start');
    coder.ceval('Model_Target_Medusa5H1Part2_Start');
    coder.ceval('Model_Target_Medusa5H1Part3_Start');

    coder.ceval('Model_Target_PreAmpPart1_Init');
    coder.ceval('Model_Target_PreAmpPart2_Init');
%     coder.ceval('Model_Target_SRCIn_Init');
%     coder.ceval('Model_Target_SRCOut_Init');
%     coder.ceval('Model_Target_AudioPilot35_Init');
    coder.ceval('Model_Target_Medusa5H1Part1_Init');
    coder.ceval('Model_Target_Medusa5H1Part2_Init');
    coder.ceval('Model_Target_Medusa5H1Part3_Init');
end

== matlab function ModelVls/InputSelect/Reset/MATLAB Function ==
  events: trigger input FUNCTION_CALL_EVENT
function fcn()

if coder.target('Rtw')
    coder.ceval('Model_Target_InputSelect_Init');
end

== matlab function ModelVls/PreAmp/DecRate/Medusa5H1/MedusaHoligram/Medusa5H1 Part 4/On/Headrest Comp EQ/FIR/FIR generic init ==
  data: u input; coeffs input; filterLengths input; inputMapping input; filterMapping input; states data_store_memory; codeWorkMemory data_store_memory; variantSelect parameter
  events: trigger input FUNCTION_CALL_EVENT
function fir_generic_init(u,coeffs, filterLengths, inputMapping, filterMapping, variantSelect)

% Generic FIR function to work with M inputs, N outputs and K filters
%
% Parameters:
%   u:              input channels [frame size x number of inputs]
%   coeffs:         coefficient sets [total filter lengths x 1]
%   filterLengths:  array of filter lengths [number of filters x 1]
%   inputMapping:   zero-based input mapping for each filter  [number of outputs x 1]
%   filterMapping:  zero-based filter mapping for each filter [number of outputs x 1]
%
% Global parameters:
%   states:         array of states [totalBufferSize x 1]
%   codeWorkMemory: working memory set up during roommode reset/init CRL
%                   function call [codeWorkMemorySize x 1]

% Extract configuration information from inputs
[frame_size, num_inputs]  = size(u);
num_outputs = numel(inputMapping);

global states;
global codeWorkMemory;

% Get the work memory and states size
workMemorySize = numel(codeWorkMemory);
statesSize = numel(states);

% Set correct data types
filter_length = uint32(filterLengths);
numCoeffSets = uint32(numel(filter_length));
frame_size = uint32(frame_size);
num_outputs = uint32(num_outputs);
num_inputs = uint32(num_inputs);
workMemorySize = uint32(workMemorySize);
statesSize = uint32(statesSize);
    
% There are three implementation types:
% Type    Value   Description
% CORE    1       Optimized assembly running on core
% ACCEL   2       Computing offloaded to accelerator peripheral
% Hexagon 3       Optimized C code running on Hexagon DSP
% GENERIC 4       Generic implementation for other targets without CRL 
%
% NOTE: GENERIC implementation does not use codeWorkMemory, thus does not
% need any custom initialization.
if (variantSelect == 1)
    y = fir_core_init(u, coeffs, states, filter_length, inputMapping, filterMapping, frame_size, numCoeffSets, num_inputs, num_outputs, codeWorkMemory);
    
    % NOTE: The CRL mechanism requires an output for the function call,
    % and appears to be optimized out if that return value isn't used. 
    % This is a dummy operation to make sure CRL ends up in generated code
    codeWorkMemory(1) = y; 
elseif (variantSelect == 2)
    y = fir_accelerator_init(u, coeffs, states, statesSize, filter_length, inputMapping, filterMapping, frame_size, ...
                             numCoeffSets, num_inputs, num_outputs, codeWorkMemory, workMemorySize);

    % NOTE: The CRL mechanism requires an output for the function call,
    % and appears to be optimized out if that return value isn't used. 
    % This is a dummy operation to make sure CRL ends up in generated code
    codeWorkMemory(1) = y; 
elseif (variantSelect == 3)
    y = fir_hexagon_init(u, coeffs, states, filter_length, inputMapping, filterMapping, frame_size, numCoeffSets, num_inputs, num_outputs, codeWorkMemory);
    
    % NOTE: The CRL mechanism requires an output for the function call,
    % and appears to be optimized out if that return value isn't used. 
    % This is a dummy operation to make sure CRL ends up in generated code
    codeWorkMemory(1) = y;

end

end


function y = fir_accelerator_init(u, coeffs, states, statesSize, filterLengths, inputMapping, filterMapping,...
                                  frameSize, numCoeffSets, numInputs, numOutputs, workMemory,...
                                  workMemorySize)                         
% If target == codegen, error out if no CRL found
coder.replace('-errorifnoreplacement');

% No init simulation code, but need to do something to ensure CRL does not
% get optimized out
y = workMemory(1) + 1;

end

function y = fir_core_init(u, coeffs, states, filterLengths, inputMapping, filterMapping,...
                             frameSize, numCoeffSets, numInputs, numOutputs, workMemory)
% If target == codegen, error out if no CRL found
coder.replace('-errorifnoreplacement');

% No init simulation code, but need to do something to ensure CRL does not
% get optimized out
y = workMemory(1) + 1;

end

function y = fir_hexagon_init(u, coeffs, states, filterLengths, inputMapping, filterMapping,...
                             frameSize, numCoeffSets, numInputs, numOutputs, workMemory)
% If target == codegen, error out if no CRL found
coder.replace('-errorifnoreplacement');

% No init simulation code, but need to do something to ensure CRL does not
% get optimized out
y = workMemory(1) + 1;

end

== matlab function ModelVls/PreAmp/DecRate/Medusa5H1/MedusaHoligram/Medusa5H1 Part 4/On/Headrest Comp EQ/FIR/ITC/init ==
  events: trigger input FUNCTION_CALL_EVENT; init output FUNCTION_CALL_EVENT
function init

init();

== matlab function ModelVls/PreAmp/DecRate/Medusa5H1/PreAmpPart2/MATLAB Function ==
  events: trigger input FUNCTION_CALL_EVENT
function fcn()

if coder.target('Rtw')
  
end

== matlab function ModelVls/PreAmp/DecRate/Medusa5H1/MedusaHoligram/Medusa5H1 Part 4/On/Headrest Comp EQ/FIR/MATLAB Function ==
  data: u input; y output; coeffs input; filterLengths input; inputMapping input; filterMapping input; states data_store_memory; variantSelect parameter; codeWorkMemory data_store_memory
function y = fir_generic(u, coeffs, filterLengths, inputMapping, filterMapping, variantSelect)
% Generic FIR function to work with M inputs, N outputs and K filters
%
% Parameters:
%   u:              input channels [frame size x number of inputs]
%   coeffs:         coefficient sets [total filter lengths x 1]
%   filterLengths:  array of filter lengths [number of filters x 1]
%   inputMapping:   zero-based input mapping for each filter  [number of outputs x 1]
%   filterMapping:  zero-based filter mapping for each filter [number of outputs x 1]
%
% Global parameters:
%   states:         array of states [totalBufferSize x 1]
%   codeWorkMemory: working memory set up during roommode reset/init CRL
%                   function call [codeWorkMemorySize x 1]

% Extract configuration information from inputs
[frame_size, num_inputs]  = size(u);
num_outputs = numel(inputMapping);

global states;
global codeWorkMemory;
    
% Set correct data types
filter_length = uint32(filterLengths);
frame_size = uint32(frame_size);
num_outputs = uint32(num_outputs);
num_inputs = uint32(num_inputs);

% Define one-frame delay buffer only for Accelerator simulation 
% Simulink will optimize this out for code generation
persistent delayedOut;
if isempty(delayedOut)
    delayedOut = single(zeros(frame_size, num_outputs));
end
    
% There are three implementation types:
% Type    Value   Description
% CORE    1       Optimized assembly running on SHARC+ core
% ACCEL   2       Computing offloaded to SHARC+ accelerator peripheral
% Hexagon 3       Optimizaed C code running on Hexagon DSP
% GENERIC 4       Generic implementation for other targets without CRL

variantSelect=4;
variantSelect

% Simulation
if(coder.target('MATLAB') || coder.target('Sfun')) 
    if (variantSelect == 2)
        % Manually insert one-frame delay in simulation to mimic 
        % Accelerator behavior
        y = delayedOut;
        delayedOut = fir_generic_simulation(u, coeffs, states, filter_length, inputMapping, ...
                filterMapping, frame_size, num_inputs, num_outputs);
    else
        y = fir_generic_simulation(u, coeffs, states, filter_length, inputMapping, ...
                filterMapping, frame_size, num_inputs, num_outputs);
    end

% Code generation
else 
    if (variantSelect == 1)
        y = fir_core_process(u, codeWorkMemory, num_outputs);
    elseif (variantSelect == 2)
        y = fir_accelerator_process(u, codeWorkMemory, num_outputs);
    elseif (variantSelect == 3)
        y = fir_hexagon_process(u, codeWorkMemory, num_outputs);        
    else
        y = fir_generic_simulation(u, coeffs, states, filter_length, inputMapping, ...
                filterMapping, frame_size, num_inputs, num_outputs);
    end  
end

end


%% CRL functions for code generation
function y = fir_core_process(u, workMemory, numOutputs)
% If target == codegen, error out if no CRL found
coder.replace('-errorifnoreplacement');
[frameSize, ~]  = size(u);
y = single(zeros(frameSize, numOutputs));
end

function y = fir_accelerator_process(u, workMemory, numOutputs)
% If target == codegen, error out if no CRL found
coder.replace('-errorifnoreplacement');
[frameSize, ~]  = size(u);
y = single(zeros(frameSize, numOutputs));
end

function y = fir_hexagon_process(u, workMemory, numOutputs)
% If target == codegen, error out if no CRL found
coder.replace('-errorifnoreplacement');
[frameSize, ~]  = size(u);
y = single(zeros(frameSize, numOutputs));
end

== matlab function ModelVls/PostProcess/Reset/MATLAB Function ==
  events: trigger input FUNCTION_CALL_EVENT
function fcn()

if coder.target('Rtw')
    coder.ceval('Model_Target_PostProcess_initialize');
    coder.ceval('Model_Target_PostProcess_Start');
    coder.ceval('Model_Target_PostProcess_Init');
end
